simulink model "xpc_dlt_p2p"  (R2013b)
settings: Solver=ode4  StartTime=0.0  StopTime=3  FixedStep=0.001  RelTol=1e-3
libraries: xpcnilib x5, xpclib x3
settings Model: BufferReuse=off  Creator=lucius  LastModifiedBy=lucius
settings OptimizationCC: BlockReduction=off  OptimizeBlockIOStorage=off  BufferReuse=off  ExpressionFolding=off  LocalBlockOutputs=off
settings HardwareCC: ProdIntDivRoundTo=Zero  ProdEndianess=LittleEndian  ProdHWDeviceType=Generic->32-bit x86 compatible
settings RTWCC: SystemTargetFile=xpctarget.tlc  TemplateMakefile=xpc_default_tmf  Description=xPC Target  ProcessScript=xpctarget_make_rtw_hook  RTWCompilerOptimization=On
settings xpcTargetCC: TargetFcnLib=ansi_tfl_table_tmw.mat  CodeReplacementLibrary=XPC_BLAS  ParMdlRefBuildCompliant=on  ConcurrentExecutionCompliant=on  CombineSignalStateStructs=off  MATLABClassNameForMDSCustomization=xpcAperiodicCustomization  GRTInterface=on  GenerateAllocFcn=off  xPCTaskExecutionProfile=off  xPCRL32EventNumber=5000  xPCLoadParamSetFile=off  xPCConcurrentTasks=off  xPCEnableSFAnimation=off

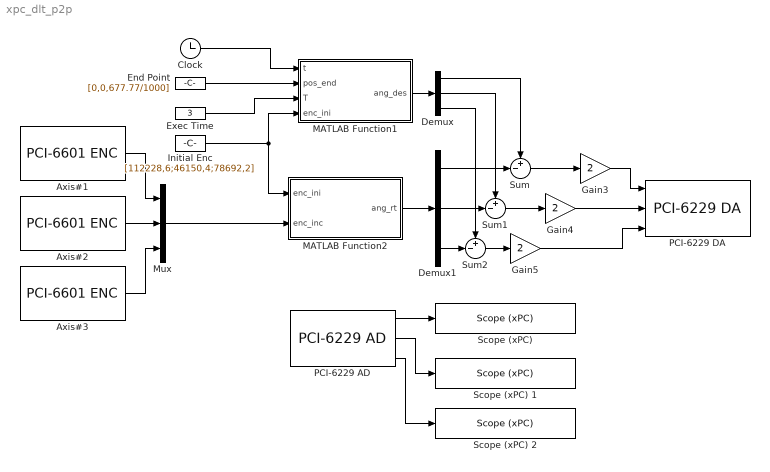
== system xpc_dlt_p2p ==
  Axis#1 : xpcnilib/Incremental Encoder/PCI-6601 ENC  channel=1  countMode=Quadrature Mode X4  initCount=0  reload=off  indexPhase=A low B low  filter=None  sampleTime=0.001  slot=-1
  Axis#2 : xpcnilib/Incremental Encoder/PCI-6601 ENC  channel=2  countMode=Quadrature Mode X4  initCount=0  reload=off  indexPhase=A low B low  filter=None  sampleTime=0.001  slot=-1
  Axis#3 : xpcnilib/Incremental Encoder/PCI-6601 ENC  channel=3  countMode=Quadrature Mode X4  initCount=0  reload=off  indexPhase=A low B low  filter=None  sampleTime=0.001  slot=-1
  Clock : Clock
  Demux : Demux  Outputs=3
  Demux1 : Demux  Outputs=3
  End Point : Constant  Value=[0,0,677.77/1000]
  Exec Time : Constant  Value=3
  Gain3 : Gain  Gain=2
  Gain4 : Gain  Gain=2
  Gain5 : Gain  Gain=2
  Initial Enc : Constant  Value=[112228,6;46150,4;78692,2]
  MATLAB Function1 : MATLAB Function  TreatAsAtomicUnit=on
  MATLAB Function2 : MATLAB Function  TreatAsAtomicUnit=on
  Mux : Mux  Inputs=3
  PCI-6229 AD : xpcnilib/A//D/M Series/PCI-6229 AD  channel=[1,3,17]  range=[10]  coupling=[0]  scantime=5e-6  sampletime=0.001  slot=-1
  PCI-6229 DA : xpcnilib/D//A/M Series/PCI-6229 DA  channel=[1,2,3]  reset=[1,1,1]  initValue=[0,0,0]  sampletime=-1  slot=-1
  "Scope (xPC) " : xpclib/Misc./Scope (xPC)   scopeno=1  scopetype=Target  autostart=on  viewmode=Graphical redraw  formatstr='%15.6f'  grid=on  ylimits=[0,0]  nosamples=250  noprepostsamples=0  interleave=1  triggermode=FreeRun  triggersignal=1  trigsignalfromport=off  triggerlevel=0.0  triggerslope=Either  triggerscope=1  triggersample=0  filename=data.dat  mode=Lazy  writesize=512  autorestart=off  dynamicfilemode=off  maxwritefilesize=512*1024^2
  Scope (xPC) 1 : xpclib/Misc./Scope (xPC)   scopeno=2  scopetype=Target  autostart=on  viewmode=Graphical redraw  formatstr='%15.6f'  grid=on  ylimits=[0,0]  nosamples=250  noprepostsamples=0  interleave=1  triggermode=FreeRun  triggersignal=1  trigsignalfromport=off  triggerlevel=0.0  triggerslope=Either  triggerscope=1  triggersample=0  filename=data.dat  mode=Lazy  writesize=512  autorestart=off  dynamicfilemode=off  maxwritefilesize=512*1024^2
  Scope (xPC) 2 : xpclib/Misc./Scope (xPC)   scopeno=3  scopetype=Target  autostart=on  viewmode=Graphical redraw  formatstr='%15.6f'  grid=on  ylimits=[0,0]  nosamples=250  noprepostsamples=0  interleave=1  triggermode=FreeRun  triggersignal=1  trigsignalfromport=off  triggerlevel=0.0  triggerslope=Either  triggerscope=1  triggersample=0  filename=data.dat  mode=Lazy  writesize=512  autorestart=off  dynamicfilemode=off  maxwritefilesize=512*1024^2
  Sum : Sum  Inputs=+-|
  Sum1 : Sum  Inputs=+-|
  Sum2 : Sum  Inputs=+-|
  wires:
  Demux/1 -> Sum/1
  Demux/3 -> Sum2/1
  Demux/2 -> Sum1/1
  Sum/1 -> Gain3/1
  Sum1/1 -> Gain4/1
  Sum2/1 -> Gain5/1
  Gain4/1 -> PCI-6229 DA/2
  Gain3/1 -> PCI-6229 DA/1
  Gain5/1 -> PCI-6229 DA/3
  PCI-6229 AD/1 -> "Scope (xPC) "/1
  PCI-6229 AD/2 -> Scope (xPC) 1/1
  PCI-6229 AD/3 -> Scope (xPC) 2/1
  Axis#1/1 -> Mux/1
  Axis#2/1 -> Mux/2
  Axis#3/1 -> Mux/3
  MATLAB Function2/1(ang_rt) -> Demux1/1
  Demux1/1 -> Sum/2
  Demux1/2 -> Sum1/2
  Demux1/3 -> Sum2/2
  Initial Enc/1 -> MATLAB Function2/1(enc_ini), MATLAB Function1/4(enc_ini)
  Clock/1 -> MATLAB Function1/1(t)
  MATLAB Function1/1(ang_des) -> Demux/1
  Mux/1 -> MATLAB Function2/2(enc_inc)
  Exec Time/1 -> MATLAB Function1/3(T)
  End Point/1 -> MATLAB Function1/2(pos_end)

== matlab function xpc_dlt_p2p/MATLAB Function1 ==
  data: t input; pos_end input; T input; enc_ini input; ang_des output
function ang_des = traj_p2p(t,pos_end,T,enc_ini)
% /***********************************************************************
% * Name:       Point to Point Trajectory of Delta Robot
% * Type:       Embedded Matlab Function
% * Author:     Yujiong Liu
% * Date:       2015.6.6
% * 
% * Input:      enc_ini     Initial absolute encoder value
% *             pos_end     Coordinate of end point
% *             t           Simulation time
% *             T           Execution time
% * 
% * Output:     ang_des     Desire joint angle
% * Function:   As shown in Name 
% ***********************************************************************/

%***********************REFERENCE****************************************
%LIMIT&ABSOLUTE NUMBER
%Axis#      Limit   Absolute Position
%1          -45     14circles   +1784
%           100     0circles    +98713

%2          -45     13circles   +120485
%           100     0circles    +87782

%3          -45     13circles   +77696
%           100     0circles    +44275

%************************COMPUTATION**************************************
%convert initial encoder value to joint angle
ang_ini=[0,0,0];
%Axis#1
ang_ini(1)=(131072*enc_ini(1,2)+enc_ini(1,1)-98713)*pi*29/36/(14*131072+1784-98713)-5*pi/9;
%Axis#2
ang_ini(2)=(131072*enc_ini(2,2)+enc_ini(2,1)-87782)*pi*29/36/(13*131072+120485-87782)-5*pi/9;
%Axis#3
ang_ini(3)=(131072*enc_ini(3,2)+enc_ini(3,1)-44275)*pi*29/36/(13*131072+77696-44275)-5*pi/9;

%convert the coordinate of the end point to joint angle by inverse
%kinematics
% PARAMETER
% /**********************************************************************/
R_B=200/1000;
L_A=270/1000;
L_F=800/1000;
R_T=45/1000;

% COMPUTATION
% /**********************************************************************/
rot_1=[1,0,0;0,1,0;0,0,1];                          %first frame
rot_2=[-0.5,-sqrt(3)/2,0;sqrt(3)/2,-0.5,0;0,0,1];   %second frame
rot_3=[-0.5,sqrt(3)/2,0;-sqrt(3)/2,-0.5,0;0,0,1];   %third frame

c_1=rot_1*[R_T;0;0]+[pos_end(1);pos_end(2);pos_end(3)];
c_2=rot_2*[R_T;0;0]+[pos_end(1);pos_end(2);pos_end(3)];
c_3=rot_3*[R_T;0;0]+[pos_end(1);pos_end(2);pos_end(3)];

a_1=rot_1*[R_B;0;0];
a_2=rot_2*[R_B;0;0];
a_3=rot_3*[R_B;0;0];

nv_1=cross(a_1',[0,0,1]);
env_1=nv_1/norm(nv_1);
lamda_1=-(env_1*c_1)/(env_1*env_1');
cp_1=lamda_1*env_1'+c_1;
acp_1=cp_1-a_1;
dis_acp_1=norm(acp_1);
%no need rotational matrix for the first one
ang_end=[0,0,0];
ang_cao_1=acos(acp_1(1)/dis_acp_1);
ang_cab_1=acos((L_A^2+dis_acp_1^2+lamda_1^2-L_F^2)/(2*L_A*dis_acp_1));
ang_end(1)=ang_cao_1-ang_cab_1;

nv_2=cross(a_2',[0,0,1]);
env_2=nv_2/norm(nv_2);
lamda_2=-(env_2*c_2)/(env_2*env_2');
cp_2=lamda_2*env_2'+c_2;
acp_2=cp_2-a_2;
dis_acp_2=norm(acp_2);
%inverse rotational matrix for the second one
rot_2_i=[-0.5,sqrt(3)/2,0;-sqrt(3)/2,-0.5,0;0,0,1];   %inverse rotation
acp_2_r=rot_2_i*acp_2;
ang_cao_2=acos(acp_2_r(1)/dis_acp_2);
ang_cab_2=acos((L_A^2+dis_acp_2^2+lamda_2^2-L_F^2)/(2*L_A*dis_acp_2));
ang_end(2)=ang_cao_2-ang_cab_2;

nv_3=cross(a_3',[0,0,1]);
env_3=nv_3/norm(nv_3);
lamda_3=-(env_3*c_3)/(env_3*env_3');
cp_3=lamda_3*env_3'+c_3;
acp_3=cp_3-a_3;
dis_acp_3=norm(acp_3);
%inverse rotational matrix for the second one
rot_3_i=[-0.5,-sqrt(3)/2,0;sqrt(3)/2,-0.5,0;0,0,1];   %inverse rotation
acp_3_r=rot_3_i*acp_3;
ang_cao_3=acos(acp_3_r(1)/dis_acp_3);
ang_cab_3=acos((L_A^2+dis_acp_3^2+lamda_3^2-L_F^2)/(2*L_A*dis_acp_3));
ang_end(3)=ang_cao_3-ang_cab_3;

%convert the kinematics angle to real angle
ang_end_r=-ang_end;

%trajectory in joint space
ang_des=[0,0,0];
ang_des(1)=(2*(ang_ini(1)-ang_end_r(1))/(T^3))*t^3+(3*(ang_end_r(1)-ang_ini(1))/(T^2))*t^2+ang_ini(1);
ang_des(2)=(2*(ang_ini(2)-ang_end_r(2))/(T^3))*t^3+(3*(ang_end_r(2)-ang_ini(2))/(T^2))*t^2+ang_ini(2);
ang_des(3)=(2*(ang_ini(3)-ang_end_r(3))/(T^3))*t^3+(3*(ang_end_r(3)-ang_ini(3))/(T^2))*t^2+ang_ini(3);

== matlab function xpc_dlt_p2p/MATLAB Function2 ==
  data: enc_ini input; ang_rt output; enc_inc input
function ang_rt = inc2jo(enc_ini,enc_inc)
%***********************REFERENCE****************************************
%LIMIT&ABSOLUTE NUMBER
%Axis#      Limit   Absolute Position
%1          -45     14circles   +1784
%           100     0circles    +98713

%2          -45     13circles   +120485
%           100     0circles    +87782

%3          -45     13circles   +77696
%           100     0circles    +44275

%************************COMPUTATION**************************************
enc_rt=[0,0,0];
enc_rt(1)=enc_ini(1,2)*131072+enc_ini(1,1)+enc_inc(1)*131072/10000;%real time
enc_rt(2)=enc_ini(2,2)*131072+enc_ini(2,1)+enc_inc(2)*131072/10000;%encoder
enc_rt(3)=enc_ini(3,2)*131072+enc_ini(3,1)+enc_inc(3)*131072/10000;%value
ang_rt=[0;0;0];
%Axis#1
ang_rt(1)=(enc_rt(1)-98713)*pi*29/36/(14*131072+1784-98713)-5*pi/9;
%Axis#2
ang_rt(2)=(enc_rt(2)-87782)*pi*29/36/(13*131072+120485-87782)-5*pi/9;
%Axis#3
ang_rt(3)=(enc_rt(3)-44275)*pi*29/36/(13*131072+77696-44275)-5*pi/9;
